simulink model "Torque_control_21b"  (R2021b)
settings: Solver=ode1  StartTime=0.0  StopTime=inf  FixedStep=0.001  RelTol=1e-3
undefined symbols (not defined in the file): a, b, D, J, k1, k2, kd4, kii, kp4, kpi, kpo, Kt, R, Tc
libraries: arduinolib x32, arduinosensorlib x7, simulink_extras x3, simulink x1
settings Model: ExtModeTrigDuration=2  Creator=LabPC  LastModifiedBy=sokse
settings OptimizationCC: EnhancedBackFolding=on  PassReuseOutputArgsAs=Individual arguments  ZeroExternalMemoryAtStartup=off  ZeroInternalMemoryAtStartup=off  MaxStackSize=64  OptimizeBlockOrder=speed  DifferentSizesBufferReuse=on  OptimizationCustomize=off  EfficientTunableParamExpr=on
settings DebuggingCC: MultiTaskRateTransMsg=warning  ParameterTunabilityLossMsg=error  UnconnectedInputMsg=none  UnconnectedOutputMsg=none  UnconnectedLineMsg=none
settings HardwareCC: ProdBitPerInt=16  ProdBitPerPointer=16  ProdBitPerSizeT=16  ProdBitPerPtrDiffT=16  ProdLargestAtomicFloat=None  ProdWordSize=8  ProdHWDeviceType=Atmel->AVR
settings SFSimCC: MATLABDynamicMemAlloc=off
settings RTWCC: Description=Embedded Coder  SystemTargetFile=ert.tlc  HardwareBoard=Arduino Mega 2560  TemplateMakefile=ert_default_tmf  Toolchain=Arduino AVR  BuildConfiguration=Faster Runs  DLArmComputeVersion=20.02.1
settings CodeAppCC: ForceParamTrailComments=on  IgnoreCustomStorageClasses=off  OperatorAnnotations=on  SimulinkDataObjDesc=on  SFDataObjDesc=on  InsertBlockDesc=on
settings ERTTargetCC: SupportContinuousTime=on  SupportVariableSizeSignals=on  ExtModeTransport=3  ExtModeStaticAlloc=on  ExtModeStaticAllocSize=2048  ExtModeMexFile=ext_xcp  ExtModeIntrfLevel=Level2 - Open

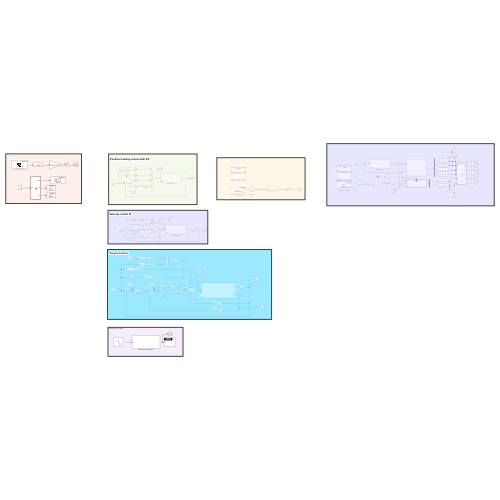
[thumbnail: Simulink's stored preview of the top-level diagram]
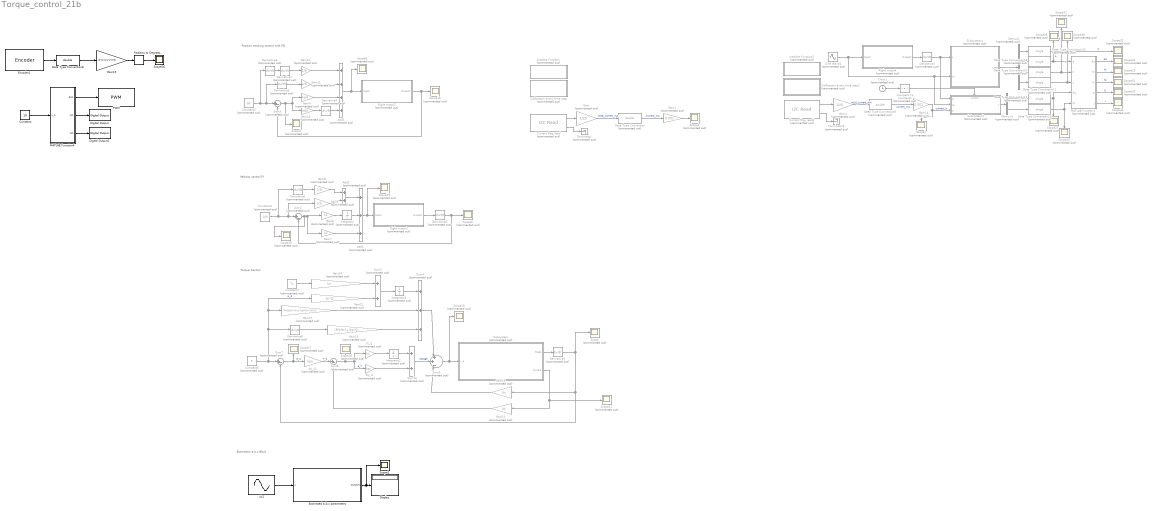
== system Torque_control_21b ==
  note: Estimation a,b,c Block
  note: Torque Control
  note: Position tracking control with PD
  note: Velocity control PI
  Add1 : Sum  Commented=on  Inputs=+++
  Add2 : Sum  Commented=on
  Add3 : Sum  Commented=on  Inputs=++++
  Calibration every time step : Subsystem  Priority=0  Commented=on
  Calibration every time step2 : Subsystem  Priority=0  Commented=on
  Clock1 : Clock  Commented=on
  Compare To Constant1 : simulink/Logic and Bit Operations/Compare To Constant  Commented=on  relop=>=  const=1  OutDataTypeStr=boolean
  Constant : Constant  Value=10
  Constant2 : Constant  Commented=on  Value=100
  Constant5 : Constant  Commented=on  Value=80
  Constant6 : Constant  Commented=on  Value=5
  Constant7 : Constant  Commented=on  Value=Tc
  Current Reg read : arduinolib/I2C Read  Commented=on  I2CModule=0  Mode=Master  SlaveAddress="hex2dec(\"0x40\")"  SlaveByteOrder=BigEndian  Direction=Receiver  RegisterAddressMode=on  RegisterAddress="hex2dec(\"0x04\")"  SlaveDataType=int16  DataLength=1  NoAck=off  RepeatedStart=off  OutputStatus=on  blockPlatform=ARDUINO  SampleTime=0.1
  Current Reg read2 : arduinolib/I2C Read  Commented=on  I2CModule=0  Mode=Master  SlaveAddress="hex2dec(\"0x40\")"  SlaveByteOrder=BigEndian  Direction=Receiver  RegisterAddressMode=on  RegisterAddress="hex2dec(\"0x04\")"  SlaveDataType=int16  DataLength=1  NoAck=off  RepeatedStart=off  OutputStatus=on  blockPlatform=ARDUINO  SampleTime=0.01
  Data Type Conversion : DataTypeConversion  Commented=on  OutDataTypeStr=double
  Data Type Conversion{10..15} (6 alike) : DataTypeConversion  Commented=on  OutDataTypeStr=single
  Data Type Conversion8 : DataTypeConversion  OutDataTypeStr=double
  Data Type Conversion9 : DataTypeConversion  Commented=on  OutDataTypeStr=double
  Demux1 : Demux  Commented=on
  Demux4 : Demux  Commented=on  Outputs=2
  Derivative{1..9} (9 alike) : Derivative  Commented=on
  Digital Output : arduinolib/Digital Output  pinNumber=11  Direction=output  blockPlatform=arduino
  Digital Output1 : arduinolib/Digital Output  pinNumber=12  Direction=output  blockPlatform=arduino
  Display : Display
  Encoder1 : arduinosensorlib/Encoder  InputA=2  InputB=3  Mode=No reset  SampleTime=-1
  Estimated a,b,c parameters : Subsystem
  Gain : Gain  Commented=on  Gain=1/25
  Gain1 : Gain  Commented=on  Gain=0.001
  Gain10 : Gain  Commented=on  Gain=kd4
  Gain11 : Gain  Commented=on  Gain=a/b
  Gain12 : Gain  Commented=on  Gain=1/b
  Gain13 : Gain  Commented=on  Gain=(R*J/Kt)+(kpi*J)
  Gain14 : Gain  Commented=on  Gain=0.001
  Gain15 : Gain  Gain=-(2*pi)/(11*4*370)
  Gain17 : Gain  Commented=on  Gain=(R*D/Kt)+Kt+(kpi*D)+(kii*J)
  Gain19 : Gain  Commented=on  Gain=Kt
  Gain21 : Gain  Commented=on  Gain=kii*D
  Gain23 : Gain  Commented=on  Gain=Kt
  Gain24 : Gain  Commented=on  Gain=kii
  Gain4 : Gain  Commented=on  Gain=1/25
  Gain5 : Gain  Commented=on  Gain=a/b
  Gain6 : Gain  Commented=on  Gain=k1
  Gain7 : Gain  Commented=on  Gain=k2
  Gain8 : Gain  Commented=on  Gain=1/b
  Gain9 : Gain  Commented=on  Gain=kp4
  Initialize Function : Subsystem  Commented=on  TreatAsAtomicUnit=on
  Initialize Function2 : Subsystem  Commented=on  TreatAsAtomicUnit=on
  Integrator : Integrator  Commented=on
  Integrator1 : Integrator  Commented=on
  Integrator2 : Integrator  Commented=on
  Ki_i2 : Gain  Commented=on  Gain=kii
  Kp_i2 : Gain  Commented=on  Gain=kpi
  Kp_o1 : Gain  Commented=on  Gain=kpo
  MATLAB Function1 : MATLAB Function  Commented=on  TreatAsAtomicUnit=on
  MATLAB Function4 : MATLAB Function  TreatAsAtomicUnit=on
  PWM : arduinolib/PWM  pinNumber=5  frequencyType=Default  desiredFrequency=490.2  achievableFrequency=490.2
  Radians to Degrees : simulink_extras/Transformations/Radians to Degrees
  Right motor2 : Subsystem  Commented=on
  Right motor3 : Subsystem  Commented=on
  Right motor4 : Subsystem  Commented=on
  Scope{,1,4,7..9,16..19,21,24..25,27..34,36..38} (24 alike) : Scope  Commented=on
  Scope2 : Scope
  Scope26 : Scope
  Sine Wave1 : Sin  Commented=on  Amplitude=12  Frequency=2*pi*1.2  SampleTime=0
  Subsystem : Subsystem  Commented=on
  Subsystem3 : Subsystem  Commented=on
  Subsystem4 : Subsystem  Commented=on
  Sum13 : Sum  Commented=on
  Sum{2..3,7..8} (4 alike) : Sum  Commented=on  Inputs=|+-
  Sum4 : Sum  Commented=on  Inputs=+++
  Sum5 : Sum  Commented=on
  Sum9 : Sum  Commented=on  Inputs=|+|+|-|
  Terminator : Terminator  Commented=on
  Terminator2 : Terminator  Commented=on
  uk2 : Sin  Amplitude=12  Frequency=2*pi*1.2  SampleTime=0
  wires:
  Estimated a,b,c parameters/1(Outport) -> Scope2/1, Display/1
  uk2/1 -> Estimated a,b,c parameters/1(u)
  Gain23/1 -> Sum8/2
  Derivative8/1 -> Gain13/1
  Sum4/1 -> Sum9/1
  Ki_i2/1 -> Integrator2/1
  Constant7/1 -> Gain24/1
  Constant6/1 -> Sum7/1, Derivative8/1, Gain17/1, Gain21/1  "w_d"
  Sum5/1 -> Integrator1/1
  Kp_o1/1 -> Sum8/1  "T_d"
  Integrator2/1 -> Sum13/1
  Gain24/1 -> Sum5/1
  Subsystem/1(Theta) -> Derivative9/1
  Sum7/1 -> Kp_o1/1, Scope17/1  "e_w"
  Sum9/1 -> Scope19/1, Subsystem/1(v_a)
  Gain17/1 -> Sum4/2
  Derivative9/1 -> Scope/1, Sum7/2, Gain19/1
  Current Reg read/1 -> Gain/1
  Data Type Conversion/1 -> Gain1/1  "current_mA"
  Sum2/1 -> Scope28/1, Gain6/1, Gain7/1
  Subsystem/2(Current) -> Gain23/1, Scope21/1
  Gain21/1 -> Sum5/2
  Derivative1/1 -> Gain8/1
  Gain5/1 -> Add2/2
  Sum8/1 -> Scope18/1, Kp_i2/1, Ki_i2/1  "e_T"
  Constant2/1 -> Gain5/1, Sum2/1, Derivative1/1
  Current Reg read/2 -> Terminator/1
  Gain19/1 -> Sum9/3
  Constant5/1 -> Derivative6/1, Derivative5/1, Sum3/1
  Right motor3/1(Outport) -> Derivative2/1
  Sum13/1 -> Sum9/2  "voltage"
  Add2/1 -> Add1/1
  Gain13/1 -> Sum4/3
  Integrator/1 -> Add1/2
  Derivative2/1 -> Scope9/1, Sum2/2
  Add1/1 -> Scope29/1, Right motor3/1(Inport)
  Gain1/1 -> Scope4/1
  Integrator1/1 -> Sum4/1
  Gain8/1 -> Add2/1
  Gain7/1 -> Add1/3
  Right motor2/1(Outport) -> Sum3/2, Scope16/1
  Gain6/1 -> Integrator/1
  Derivative4/1 -> Add3/4
  Kp_i2/1 -> Sum13/2
  Derivative6/1 -> Derivative7/1
  Sum3/1 -> Scope7/1, Gain9/1, Gain10/1
  Gain/1 -> Data Type Conversion/1  "int16_current_mA"
  Derivative5/1 -> Gain11/1
  Gain12/1 -> Add3/1
  Gain10/1 -> Derivative4/1
  Gain11/1 -> Add3/2
  Derivative7/1 -> Gain12/1
  Gain9/1 -> Add3/3
  Add3/1 -> Scope8/1, Right motor2/1(Inport)
  Radians to Degrees/1 -> Scope26/1
  Gain15/1 -> Radians to Degrees/1
  Data Type Conversion8/1 -> Gain15/1
  Encoder1/1 -> Data Type Conversion8/1
  MATLAB Function1/5(J) -> Scope34/1  "J"
  MATLAB Function1/2(kt) -> Scope25/1  "kt"
  Gain4/1 -> Data Type Conversion9/1  "int16_current_mA"
  Gain14/1 -> Scope1/1, Subsystem3/3(ci)  "current_A"
  Demux1/2 -> Data Type Conversion14/1
  Demux4/1 -> Data Type Conversion12/1
  Sine Wave1/1 -> Right motor4/1(Inport), Subsystem3/2(va), Subsystem4/2(uk)
  Current Reg read2/1 -> Gain4/1
  Data Type Conversion9/1 -> Gain14/1  "current_mA"
  Demux1/3 -> Data Type Conversion10/1
  MATLAB Function1/1(Ra) -> Scope24/1  "Ra"
  Demux4/2 -> Data Type Conversion13/1
  Subsystem3/1(x) -> Demux4/1
  Data Type Conversion10/1 -> Scope37/1, MATLAB Function1/2(b)  "b"
  Demux1/1 -> Data Type Conversion15/1
  Data Type Conversion14/1 -> MATLAB Function1/1(a), Scope36/1  "a"
  Data Type Conversion15/1 -> Scope32/1  "w"
  Subsystem4/1(x_est) -> Demux1/1
  Right motor4/1(Outport) -> Derivative3/1
  Derivative3/1 -> Subsystem3/1(w), Subsystem4/1(x)
  Current Reg read2/2 -> Terminator2/1
  Data Type Conversion11/1 -> Scope38/1, MATLAB Function1/3(c)  "c"
  MATLAB Function1/3(Tc) -> Scope31/1  "Tc"
  Demux1/4 -> Data Type Conversion11/1
  Data Type Conversion12/1 -> MATLAB Function1/4("Ra "), Scope27/1
  Data Type Conversion13/1 -> MATLAB Function1/5("kt "), Scope30/1
  MATLAB Function1/4(D) -> Scope33/1  "D"
  Compare To Constant1/1 -> Subsystem3/Enable
  Clock1/1 -> Compare To Constant1/1
  MATLAB Function4/2(IN1) -> Digital Output/1
  Constant/1 -> MATLAB Function4/1(v_a)
  MATLAB Function4/1(ENA) -> PWM/1
  MATLAB Function4/3(IN2) -> Digital Output1/1

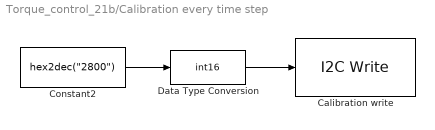
== system Torque_control_21b/Calibration every time step ==
  Calibration write : arduinolib/I2C Write  I2CModule=0  Mode=Master  SlaveAddress="uint8(hex2dec(\"0x40\"))"  SlaveByteOrder=BigEndian  Direction=Transmitter  RegisterAddressMode=on  RegisterAddress="uint8(hex2dec(\"0x05\"))"  SlaveDataType=uint8  DataLength=1  NoAck=off  RepeatedStart=off  OutputStatus=off  blockPlatform=ARDUINO
  Constant2 : Constant  Value="hex2dec(\"2800\")"
  Data Type Conversion : DataTypeConversion  OutDataTypeStr=int16
  wires:
  Constant2/1 -> Data Type Conversion/1
  Data Type Conversion/1 -> Calibration write/1

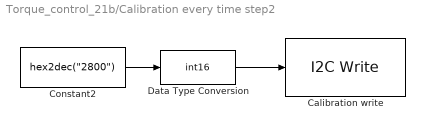
== system Torque_control_21b/Calibration every time step2 ==
  Calibration write : arduinolib/I2C Write  I2CModule=0  Mode=Master  SlaveAddress="uint8(hex2dec(\"0x40\"))"  SlaveByteOrder=BigEndian  Direction=Transmitter  RegisterAddressMode=on  RegisterAddress="uint8(hex2dec(\"0x05\"))"  SlaveDataType=uint8  DataLength=1  NoAck=off  RepeatedStart=off  OutputStatus=off  blockPlatform=ARDUINO
  Constant2 : Constant  Value="hex2dec(\"2800\")"
  Data Type Conversion : DataTypeConversion  OutDataTypeStr=int16
  wires:
  Constant2/1 -> Data Type Conversion/1
  Data Type Conversion/1 -> Calibration write/1

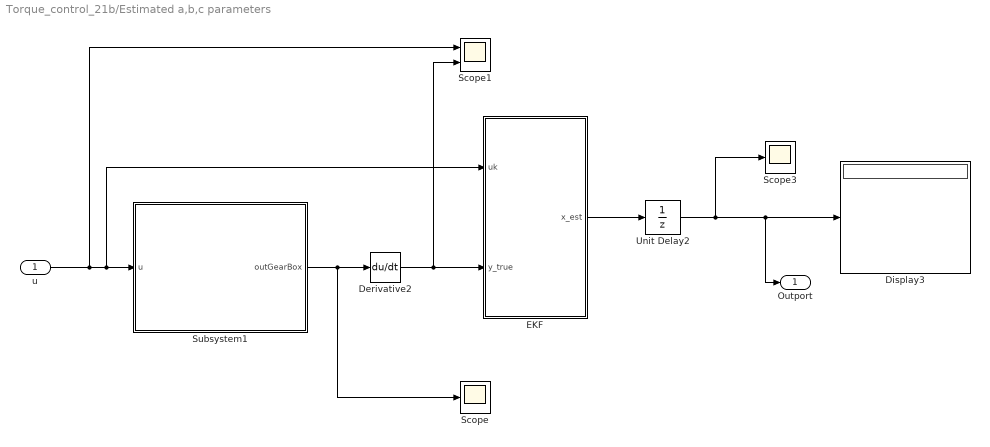
== system Torque_control_21b/Estimated a,b,c parameters ==
  u : Inport
  Derivative2 : Derivative
  Display3 : Display
  EKF : MATLAB Function  TreatAsAtomicUnit=on
  Scope : Scope
  Scope1 : Scope  NumInputPorts=2
  Scope3 : Scope
  Subsystem1 : Subsystem
  Unit Delay2 : UnitDelay  InitialCondition=[0;0;0;0]  SampleTime=-1  HasFrameUpgradeWarning=on
  Outport : Outport
  wires:
  Derivative2/1 -> Scope1/2, EKF/2(y_true)
  Unit Delay2/1 -> Outport/1, Display3/1, Scope3/1
  EKF/1(x_est) -> Unit Delay2/1
  Subsystem1/1(outGearBox) -> Scope/1, Derivative2/1
  u/1 -> Scope1/1, EKF/1(uk), Subsystem1/1(u)

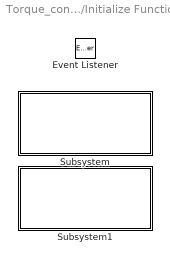
== system Torque_control_21b/Initialize Function ==
  Event Listener : EventListener  DisableCoverage=on  EventName=reset
  Subsystem : Subsystem  Priority=0
  Subsystem1 : Subsystem  Priority=1

== system Torque_control_21b/Initialize Function2 ==
  Event Listener : EventListener  DisableCoverage=on  EventName=reset
  Subsystem : Subsystem  Priority=0
  Subsystem1 : Subsystem  Priority=1

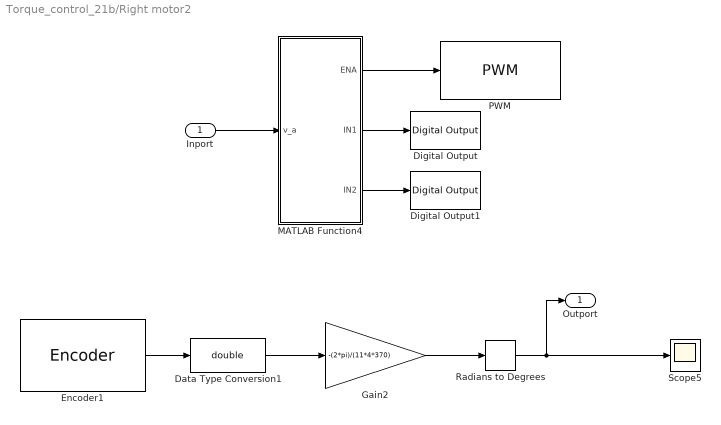
== system Torque_control_21b/Right motor2 ==
  Inport : Inport
  Data Type Conversion1 : DataTypeConversion  OutDataTypeStr=double
  Digital Output : arduinolib/Digital Output  pinNumber=5  Direction=output  blockPlatform=arduino
  Digital Output1 : arduinolib/Digital Output  pinNumber=7  Direction=output  blockPlatform=arduino
  Encoder1 : arduinosensorlib/Encoder  InputA=2  InputB=3  Mode=No reset  SampleTime=0.001
  Gain2 : Gain  Gain=-(2*pi)/(11*4*370)
  MATLAB Function4 : MATLAB Function  TreatAsAtomicUnit=on
  PWM : arduinolib/PWM  pinNumber=4  frequencyType=Default  desiredFrequency=490.2  achievableFrequency=490.2
  Radians to Degrees : simulink_extras/Transformations/Radians to Degrees
  Scope5 : Scope
  Outport : Outport
  wires:
  Gain2/1 -> Radians to Degrees/1
  Data Type Conversion1/1 -> Gain2/1
  Encoder1/1 -> Data Type Conversion1/1
  MATLAB Function4/1(ENA) -> PWM/1
  MATLAB Function4/2(IN1) -> Digital Output/1
  MATLAB Function4/3(IN2) -> Digital Output1/1
  Inport/1 -> MATLAB Function4/1(v_a)
  Radians to Degrees/1 -> Outport/1, Scope5/1

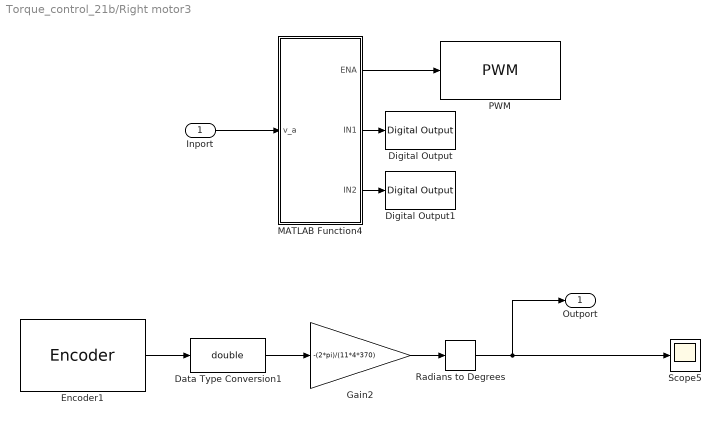
== system Torque_control_21b/Right motor3 ==
  Inport : Inport
  Data Type Conversion1 : DataTypeConversion  OutDataTypeStr=double
  Digital Output : arduinolib/Digital Output  pinNumber=5  Direction=output  blockPlatform=arduino
  Digital Output1 : arduinolib/Digital Output  pinNumber=7  Direction=output  blockPlatform=arduino
  Encoder1 : arduinosensorlib/Encoder  InputA=2  InputB=3  Mode=No reset  SampleTime=0.001
  Gain2 : Gain  Gain=-(2*pi)/(11*4*370)
  MATLAB Function4 : MATLAB Function  TreatAsAtomicUnit=on
  PWM : arduinolib/PWM  pinNumber=4  frequencyType=Default  desiredFrequency=490.2  achievableFrequency=490.2
  Radians to Degrees : simulink_extras/Transformations/Radians to Degrees
  Scope5 : Scope
  Outport : Outport
  wires:
  Radians to Degrees/1 -> Scope5/1, Outport/1
  Inport/1 -> MATLAB Function4/1(v_a)
  MATLAB Function4/3(IN2) -> Digital Output1/1
  MATLAB Function4/2(IN1) -> Digital Output/1
  MATLAB Function4/1(ENA) -> PWM/1
  Encoder1/1 -> Data Type Conversion1/1
  Data Type Conversion1/1 -> Gain2/1
  Gain2/1 -> Radians to Degrees/1

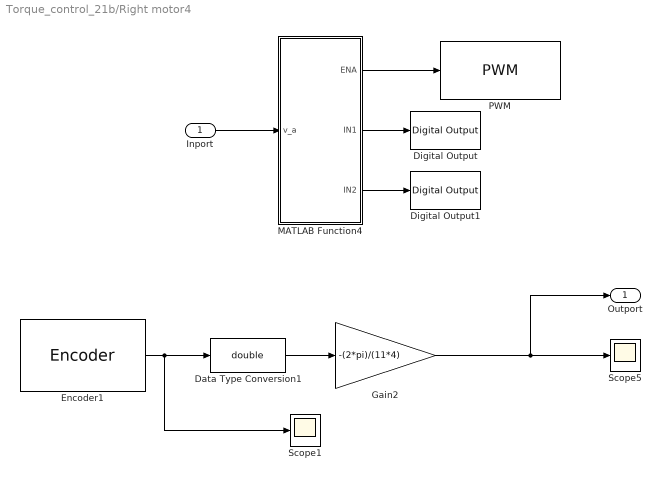
== system Torque_control_21b/Right motor4 ==
  Inport : Inport
  Data Type Conversion1 : DataTypeConversion  OutDataTypeStr=double
  Digital Output : arduinolib/Digital Output  pinNumber=5  Direction=output  blockPlatform=arduino
  Digital Output1 : arduinolib/Digital Output  pinNumber=7  Direction=output  blockPlatform=arduino
  Encoder1 : arduinosensorlib/Encoder  InputA=2  InputB=3  Mode=No reset  SampleTime=0.01
  Gain2 : Gain  Gain=-(2*pi)/(11*4)
  MATLAB Function4 : MATLAB Function  TreatAsAtomicUnit=on
  PWM : arduinolib/PWM  pinNumber=4  frequencyType=Default  desiredFrequency=490.2  achievableFrequency=490.2
  Scope1 : Scope
  Scope5 : Scope
  Outport : Outport
  wires:
  Data Type Conversion1/1 -> Gain2/1
  Encoder1/1 -> Scope1/1, Data Type Conversion1/1
  MATLAB Function4/3(IN2) -> Digital Output1/1
  Inport/1 -> MATLAB Function4/1(v_a)
  MATLAB Function4/1(ENA) -> PWM/1
  MATLAB Function4/2(IN1) -> Digital Output/1
  Gain2/1 -> Outport/1, Scope5/1

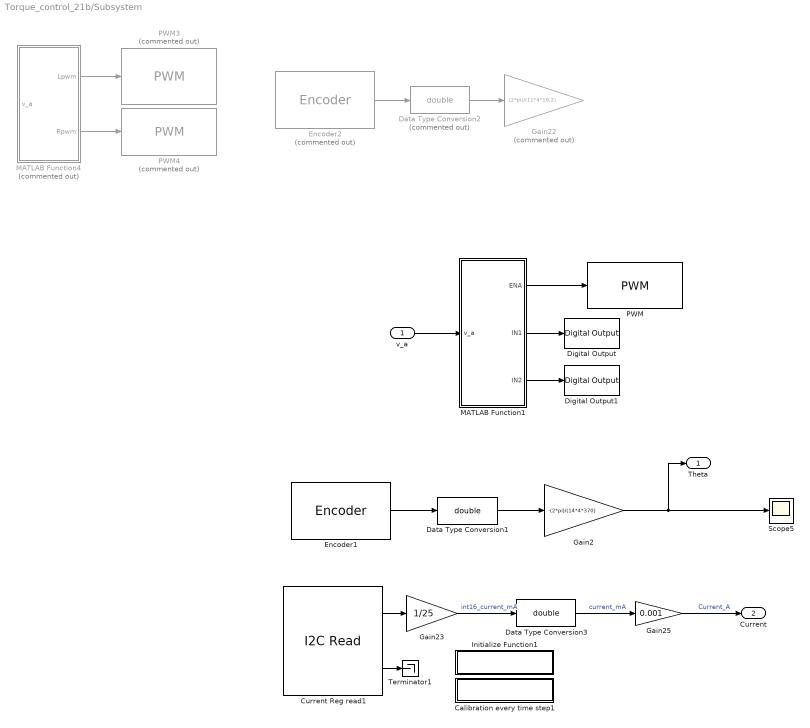
== system Torque_control_21b/Subsystem ==
  v_a : Inport
  Calibration every time step1 : Subsystem  Priority=0
  Current Reg read1 : arduinolib/I2C Read  I2CModule=0  Mode=Master  SlaveAddress="hex2dec(\"0x40\")"  SlaveByteOrder=BigEndian  Direction=Receiver  RegisterAddressMode=on  RegisterAddress="hex2dec(\"0x04\")"  SlaveDataType=int16  DataLength=1  NoAck=off  RepeatedStart=off  OutputStatus=on  blockPlatform=ARDUINO  SampleTime=0.1
  Data Type Conversion1 : DataTypeConversion  OutDataTypeStr=double
  Data Type Conversion2 : DataTypeConversion  Commented=on  OutDataTypeStr=double
  Data Type Conversion3 : DataTypeConversion  OutDataTypeStr=double
  Digital Output : arduinolib/Digital Output  pinNumber=5  Direction=output  blockPlatform=arduino
  Digital Output1 : arduinolib/Digital Output  pinNumber=7  Direction=output  blockPlatform=arduino
  Encoder1 : arduinosensorlib/Encoder  InputA=2  InputB=3  Mode=No reset  SampleTime=-1
  Encoder2 : arduinosensorlib/Encoder  Commented=on  InputA=2  InputB=3  Mode=No reset  SampleTime=-1
  Gain2 : Gain  Gain=-(2*pi)/(14*4*370)
  Gain22 : Gain  Commented=on  Gain=(2*pi)/(11*4*19.2)
  Gain23 : Gain  Gain=1/25
  Gain25 : Gain  Gain=0.001
  Initialize Function1 : Subsystem  TreatAsAtomicUnit=on
  MATLAB Function1 : MATLAB Function  TreatAsAtomicUnit=on
  MATLAB Function4 : MATLAB Function  Commented=on  TreatAsAtomicUnit=on
  PWM : arduinolib/PWM  pinNumber=4  frequencyType=Default  desiredFrequency=490.2  achievableFrequency=490.2
  PWM3 : arduinolib/PWM  Commented=on  pinNumber=8  frequencyType=Default  desiredFrequency=490.2  achievableFrequency=490.2
  PWM4 : arduinolib/PWM  Commented=on  pinNumber=9  frequencyType=Default  desiredFrequency=490.2  achievableFrequency=490.2
  Scope5 : Scope
  Terminator1 : Terminator
  Theta : Outport
  Current : Outport  Port=2
  wires:
  Current Reg read1/2 -> Terminator1/1
  Data Type Conversion3/1 -> Gain25/1  "current_mA"
  Gain23/1 -> Data Type Conversion3/1  "int16_current_mA"
  Data Type Conversion2/1 -> Gain22/1
  Encoder2/1 -> Data Type Conversion2/1
  MATLAB Function4/1(Lpwm) -> PWM3/1
  MATLAB Function4/2(Rpwm) -> PWM4/1
  Current Reg read1/1 -> Gain23/1
  Gain25/1 -> Current/1  "Current_A"
  Gain2/1 -> Theta/1, Scope5/1
  MATLAB Function1/1(ENA) -> PWM/1
  Data Type Conversion1/1 -> Gain2/1
  Encoder1/1 -> Data Type Conversion1/1
  MATLAB Function1/3(IN2) -> Digital Output1/1
  MATLAB Function1/2(IN1) -> Digital Output/1
  v_a/1 -> MATLAB Function1/1(v_a)

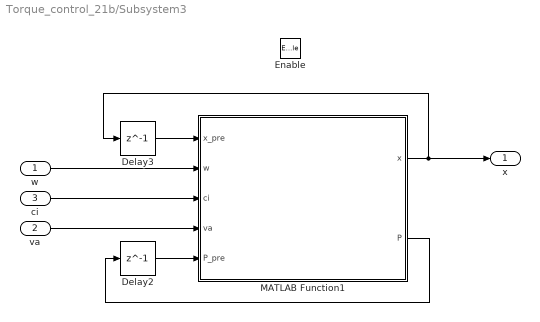
== system Torque_control_21b/Subsystem3 ==
  w : Inport
  va : Inport  Port=2
  ci : Inport  Port=3
  Enable : EnablePort
  Delay2 : Delay  DelayLength=1  InitialCondition=diag([5,0.1])
  Delay3 : Delay  DelayLength=1  InitialCondition=[5;0.4]
  MATLAB Function1 : MATLAB Function  TreatAsAtomicUnit=on
  x : Outport
  wires:
  MATLAB Function1/1(x) -> x/1, Delay3/1
  Delay2/1 -> MATLAB Function1/5(P_pre)
  MATLAB Function1/2(P) -> Delay2/1
  Delay3/1 -> MATLAB Function1/1(x_pre)
  ci/1 -> MATLAB Function1/3(ci)
  w/1 -> MATLAB Function1/2(w)
  va/1 -> MATLAB Function1/4(va)

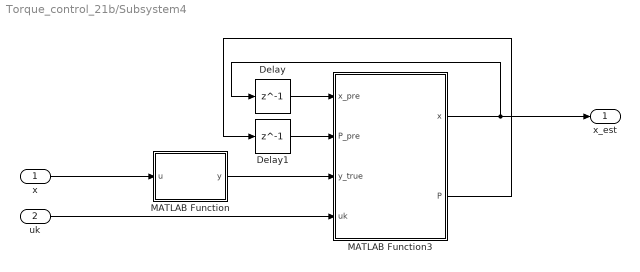
== system Torque_control_21b/Subsystem4 ==
  x : Inport
  uk : Inport  Port=2
  Delay : Delay  DelayLength=1  InitialCondition=[0;0;0;0]
  Delay1 : Delay  DelayLength=1  InitialCondition=1e0*diag([10,1,30,10])
  MATLAB Function : MATLAB Function  TreatAsAtomicUnit=on
  MATLAB Function3 : MATLAB Function  TreatAsAtomicUnit=on
  x_est : Outport
  wires:
  x/1 -> MATLAB Function/1(u)
  Delay/1 -> MATLAB Function3/1(x_pre)
  Delay1/1 -> MATLAB Function3/2(P_pre)
  MATLAB Function3/2(P) -> Delay1/1
  uk/1 -> MATLAB Function3/4(uk)
  MATLAB Function3/1(x) -> Delay/1, x_est/1
  MATLAB Function/1(y) -> MATLAB Function3/3(y_true)

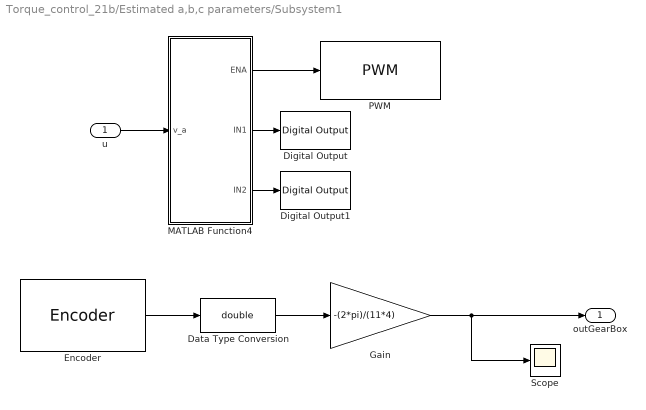
== system Torque_control_21b/Estimated a,b,c parameters/Subsystem1 ==
  u : Inport
  Data Type Conversion : DataTypeConversion  OutDataTypeStr=double
  Digital Output : arduinolib/Digital Output  pinNumber=11  Direction=output  blockPlatform=arduino
  Digital Output1 : arduinolib/Digital Output  pinNumber=12  Direction=output  blockPlatform=arduino
  Encoder : arduinosensorlib/Encoder  InputA=2  InputB=3  Mode=No reset  SampleTime=-1
  Gain : Gain  Gain=-(2*pi)/(11*4)
  MATLAB Function4 : MATLAB Function  TreatAsAtomicUnit=on
  PWM : arduinolib/PWM  pinNumber=5  frequencyType=Default  desiredFrequency=490.2  achievableFrequency=490.2
  Scope : Scope
  outGearBox : Outport
  wires:
  Gain/1 -> Scope/1, outGearBox/1
  Encoder/1 -> Data Type Conversion/1
  Data Type Conversion/1 -> Gain/1
  MATLAB Function4/2(IN1) -> Digital Output/1
  MATLAB Function4/1(ENA) -> PWM/1
  MATLAB Function4/3(IN2) -> Digital Output1/1
  u/1 -> MATLAB Function4/1(v_a)

== system Torque_control_21b/Initialize Function/Subsystem ==
  Configuration write : arduinolib/I2C Write  I2CModule=0  Mode=Master  SlaveAddress="hex2dec(\"0x40\")"  SlaveByteOrder=BigEndian  Direction=Transmitter  RegisterAddressMode=on  RegisterAddress="hex2dec(\"0x00\")"  SlaveDataType=uint8  DataLength=1  NoAck=off  RepeatedStart=off  OutputStatus=off  blockPlatform=ARDUINO
  Constant3 : Constant  Value="hex2dec(\"399F\")"
  Data Type Conversion : DataTypeConversion  OutDataTypeStr=int16
  wires:
  Constant3/1 -> Data Type Conversion/1
  Data Type Conversion/1 -> Configuration write/1

== system Torque_control_21b/Initialize Function/Subsystem1 ==
  Calibration write : arduinolib/I2C Write  I2CModule=0  Mode=Master  SlaveAddress="uint8(hex2dec(\"0x40\"))"  SlaveByteOrder=BigEndian  Direction=Transmitter  RegisterAddressMode=on  RegisterAddress="uint8(hex2dec(\"0x05\"))"  SlaveDataType=uint8  DataLength=1  NoAck=off  RepeatedStart=off  OutputStatus=off  blockPlatform=ARDUINO
  Constant2 : Constant  Value="hex2dec(\"0x2800\")"
  Data Type Conversion : DataTypeConversion  OutDataTypeStr=int16
  wires:
  Constant2/1 -> Data Type Conversion/1
  Data Type Conversion/1 -> Calibration write/1

== system Torque_control_21b/Initialize Function2/Subsystem ==
  Configuration write : arduinolib/I2C Write  I2CModule=0  Mode=Master  SlaveAddress="hex2dec(\"0x40\")"  SlaveByteOrder=BigEndian  Direction=Transmitter  RegisterAddressMode=on  RegisterAddress="hex2dec(\"0x00\")"  SlaveDataType=uint8  DataLength=1  NoAck=off  RepeatedStart=off  OutputStatus=off  blockPlatform=ARDUINO
  Constant3 : Constant  Value="hex2dec(\"399F\")"
  Data Type Conversion : DataTypeConversion  OutDataTypeStr=int16
  wires:
  Constant3/1 -> Data Type Conversion/1
  Data Type Conversion/1 -> Configuration write/1

== system Torque_control_21b/Initialize Function2/Subsystem1 ==
  Calibration write : arduinolib/I2C Write  I2CModule=0  Mode=Master  SlaveAddress="uint8(hex2dec(\"0x40\"))"  SlaveByteOrder=BigEndian  Direction=Transmitter  RegisterAddressMode=on  RegisterAddress="uint8(hex2dec(\"0x05\"))"  SlaveDataType=uint8  DataLength=1  NoAck=off  RepeatedStart=off  OutputStatus=off  blockPlatform=ARDUINO
  Constant2 : Constant  Value="hex2dec(\"0x2800\")"
  Data Type Conversion : DataTypeConversion  OutDataTypeStr=int16
  wires:
  Constant2/1 -> Data Type Conversion/1
  Data Type Conversion/1 -> Calibration write/1

== system Torque_control_21b/Subsystem/Calibration every time step1 ==
  Calibration write : arduinolib/I2C Write  I2CModule=0  Mode=Master  SlaveAddress="uint8(hex2dec(\"0x40\"))"  SlaveByteOrder=BigEndian  Direction=Transmitter  RegisterAddressMode=on  RegisterAddress="uint8(hex2dec(\"0x05\"))"  SlaveDataType=uint8  DataLength=1  NoAck=off  RepeatedStart=off  OutputStatus=off  blockPlatform=ARDUINO
  Constant2 : Constant  Value="hex2dec(\"2800\")"
  Data Type Conversion : DataTypeConversion  OutDataTypeStr=int16
  wires:
  Data Type Conversion/1 -> Calibration write/1
  Constant2/1 -> Data Type Conversion/1

== system Torque_control_21b/Subsystem/Initialize Function1 ==
  Event Listener : EventListener  DisableCoverage=on  EventName=reset
  Subsystem : Subsystem  Priority=0
  Subsystem1 : Subsystem  Priority=1

== system Torque_control_21b/Subsystem/Initialize Function1/Subsystem ==
  Configuration write : arduinolib/I2C Write  I2CModule=0  Mode=Master  SlaveAddress="hex2dec(\"0x40\")"  SlaveByteOrder=BigEndian  Direction=Transmitter  RegisterAddressMode=on  RegisterAddress="hex2dec(\"0x00\")"  SlaveDataType=uint8  DataLength=1  NoAck=off  RepeatedStart=off  OutputStatus=off  blockPlatform=ARDUINO
  Constant3 : Constant  Value="hex2dec(\"399F\")"
  Data Type Conversion : DataTypeConversion  OutDataTypeStr=int16
  wires:
  Data Type Conversion/1 -> Configuration write/1
  Constant3/1 -> Data Type Conversion/1

== system Torque_control_21b/Subsystem/Initialize Function1/Subsystem1 ==
  Calibration write : arduinolib/I2C Write  I2CModule=0  Mode=Master  SlaveAddress="uint8(hex2dec(\"0x40\"))"  SlaveByteOrder=BigEndian  Direction=Transmitter  RegisterAddressMode=on  RegisterAddress="uint8(hex2dec(\"0x05\"))"  SlaveDataType=uint8  DataLength=1  NoAck=off  RepeatedStart=off  OutputStatus=off  blockPlatform=ARDUINO
  Constant2 : Constant  Value="hex2dec(\"0x2800\")"
  Data Type Conversion : DataTypeConversion  OutDataTypeStr=int16
  wires:
  Data Type Conversion/1 -> Calibration write/1
  Constant2/1 -> Data Type Conversion/1

== matlab function Torque_control_21b/Right motor4/MATLAB Function4 ==
  data: v_a input; ENA output; IN1 output; IN2 output
function [ENA,IN1,IN2] = fcn(v_a)

vmax = 12;
pwm_cal = v_a*254/vmax;

if pwm_cal > 0
   
    ENA = pwm_cal;
    IN1 = 1;
    IN2 = 0;
elseif pwm_cal < 0
   
    ENA = abs(pwm_cal);
    IN1 = 0;
    IN2 = 1;
else
    ENA = 0;
    IN1 = 0;
    IN2 = 0;
   
end

== matlab function Torque_control_21b/Subsystem3/MATLAB Function1 ==
  data: x_pre input; w input; ci input; va input; P_pre input; x output; P output
function [x,P] = fcn(x_pre,w,ci,va,P_pre)
% Initialize step, putted in the delay instead
% P = (A'A)^-1;
% x = P*(A'b);

% calculate state
A = [ci w];

% recursive least square method
P = P_pre - P_pre*A'/(1+A*P_pre*A')*(A*P_pre);
K = P*A';
x = x_pre + K*(va-A*x_pre);

== matlab function Torque_control_21b/Subsystem4/MATLAB Function ==
  data: u input; y output
function y = fcn(u)

y = u(1);

== matlab function Torque_control_21b/Subsystem4/MATLAB Function3 ==
  settings: updateMethod=DISCRETE
  data: x_pre input; P_pre input; y_true input; x output; uk input; P output
function [x,P] = ekf(x_pre,P_pre,y_true, uk)
Ts = 0.01;

Qc_est  = 1e-4*diag([1,10,100,10]);
Qd_est  = Ts*Qc_est;
R_est   = 0.01;

Ck = [1 0 0 0];
Dk = 0;


% PREDICTION STEP
%Compute prediction at next time step
x = x_pre+Ts*[-x_pre(2)*x_pre(1) + uk*x_pre(3) - x_pre(4)*sign(x_pre(1));
                0;
                0;
                0];

Ak = eye(4)+Ts*[-x_pre(2) -x_pre(1) uk -sign(x_pre(1));
                 0     0    0      0;
                 0     0    0      0;
                 0     0    0      0];
P = Ak*P_pre*Ak'+Qd_est;

% OBSERVATION AND UPDATE
%Comput Kalman Gain and update predicted value
Wk    = P*Ck'/(Ck*P*Ck'+R_est);
y_est = Ck*x+Dk*uk;
dely = y_true-y_est;
Wkdely = Wk*dely;
x = x+Wkdely;
P = P-Wk*Ck*P;

== matlab function Torque_control_21b/Right motor3/MATLAB Function4 ==
  data: v_a input; ENA output; IN1 output; IN2 output
function [ENA,IN1,IN2] = fcn(v_a)

vmax = 12;
pwm_cal = v_a*254/vmax;

if pwm_cal > 0
   
    ENA = pwm_cal;
    IN1 = 1;
    IN2 = 0;
elseif pwm_cal < 0
   
    ENA = abs(pwm_cal);
    IN1 = 0;
    IN2 = 1;
else
    ENA = 0;
    IN1 = 0;
    IN2 = 0;
   
end

== matlab function Torque_control_21b/Subsystem/MATLAB Function1 ==
  data: v_a input; ENA output; IN1 output; IN2 output
function [ENA,IN1,IN2] = fcn(v_a)

vmax = 12;
pwm_cal = v_a*254/vmax;

if pwm_cal > 0
   
    ENA = pwm_cal;
    IN1 = 1;
    IN2 = 0;
elseif pwm_cal < 0
   
    ENA = abs(pwm_cal);
    IN1 = 0;
    IN2 = 1;
else
    ENA = 0;
    IN1 = 0;
    IN2 = 0;
   
end

== matlab function Torque_control_21b/Estimated a,b,c parameters/EKF ==
  settings: updateMethod=DISCRETE
  data: uk input; y_true input; x_est output
function x_est = fcn(uk,y_true)
Ts=0.01;
persistent x_est_p P Qd_est R_est Qc_est;
if isempty(x_est_p)
          
          x_est_p=[2;16;3.5;2];
          P=2*eye(4);
         Qc_est=1e-3*diag([10,10,10,1]);
          Qd_est=Qc_est*Ts;
          R_est=0.02;
end
c=[1 0 0 0];D=0;Ck=c;Dk=D;
%Comput Kalman Gain and update predicted value
Wk=P*Ck'/(Ck*P*Ck'+R_est);
y_est=Ck*x_est_p+Dk*uk;
x=x_est_p+Wk.*(y_true-y_est);
%Compute prediction at next time step
x_est=x+Ts*[-x(2)*x(1)+uk*x(3)-x(4)*sign(x(1));0;0;0];
%Update error covariance matrices
P=P-Wk*Ck*P;
%Define Ak
Ak=eye(4)+Ts*[-x(2) -x(1) uk -sign(x(1));0 0 0 0;0 0 0 0;0 0 0 0];
P=Ak*P*Ak'+Qd_est;
x_est_p=x_est;

== matlab function Torque_control_21b/Estimated a,b,c parameters/Subsystem1/MATLAB Function4 ==
  data: v_a input; ENA output; IN1 output; IN2 output
function [ENA,IN1,IN2] = fcn(v_a)

vmax = 12;
pwm_cal = v_a*254/vmax;

if pwm_cal > 0
   
    ENA = pwm_cal;
    IN1 = 1;
    IN2 = 0;
elseif pwm_cal < 0
   
    ENA = abs(pwm_cal);
    IN1 = 0;
    IN2 = 1;
else
    ENA = 0;
    IN1 = 0;
    IN2 = 0;
   
end

== matlab function Torque_control_21b/MATLAB Function4 ==
  data: v_a input; ENA output; IN1 output; IN2 output
function [ENA,IN1,IN2] = fcn(v_a)

vmax = 12;
pwm_cal = v_a*254/vmax;

if pwm_cal > 0
   
    ENA = pwm_cal;
    IN1 = 1;
    IN2 = 0;
elseif pwm_cal < 0
   
    ENA = abs(pwm_cal);
    IN1 = 0;
    IN2 = 1;
else
    ENA = 0;
    IN1 = 0;
    IN2 = 0;
   
end

== matlab function Torque_control_21b/Subsystem/MATLAB Function4 ==
  data: v_a input; Lpwm output; Rpwm output
function [Lpwm,Rpwm] = fcn(v_a)

vmax = 22.9;
pwm_cal = v_a*254/vmax;

if pwm_cal > 0
    Lpwm = 0;
    Rpwm = pwm_cal;
elseif pwm_cal < 0
    Lpwm = abs(pwm_cal);
    Rpwm = 0;
else
    Lpwm = 0;
    Rpwm = 0;
end

== matlab function Torque_control_21b/Right motor2/MATLAB Function4 ==
  data: v_a input; ENA output; IN1 output; IN2 output
function [ENA,IN1,IN2] = fcn(v_a)

vmax = 12;
pwm_cal = v_a*254/vmax;

if pwm_cal > 0
   
    ENA = pwm_cal;
    IN1 = 1;
    IN2 = 0;
elseif pwm_cal < 0
   
    ENA = abs(pwm_cal);
    IN1 = 0;
    IN2 = 1;
else
    ENA = 0;
    IN1 = 0;
    IN2 = 0;
   
end

== matlab function Torque_control_21b/MATLAB Function1 ==
  data: Ra output; kt output; Tc output; D output; a input; b input; c input; Ra input; J output; kt input
function [Ra,kt,Tc, D, J] = fcn(a, b, c, Ra, kt)
Ra = Ra;
kt = kt;

J = (kt/(Ra*b));
Tc = (c*J);
D = (a*Ra*J - kt^2)/Ra;
